simulink model "CS_SKILL_5_TDM"  (R2024a)
settings: Solver=VariableStepAuto  StartTime=0.0  StopTime=10.0  RelTol=1e-3
model workspace (MAT data in the model file):
  pi = 2
libraries: dspfdesign x3
settings Model: Creator=dev22  LastModifiedBy=dev22
settings RTWCC: GPUComputeCapability=3.5

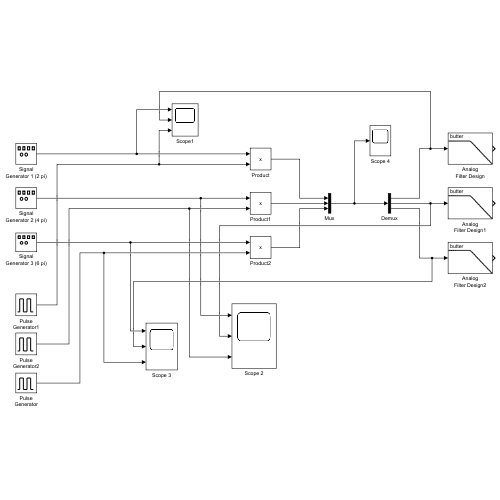
[thumbnail: Simulink's stored preview of the top-level diagram]
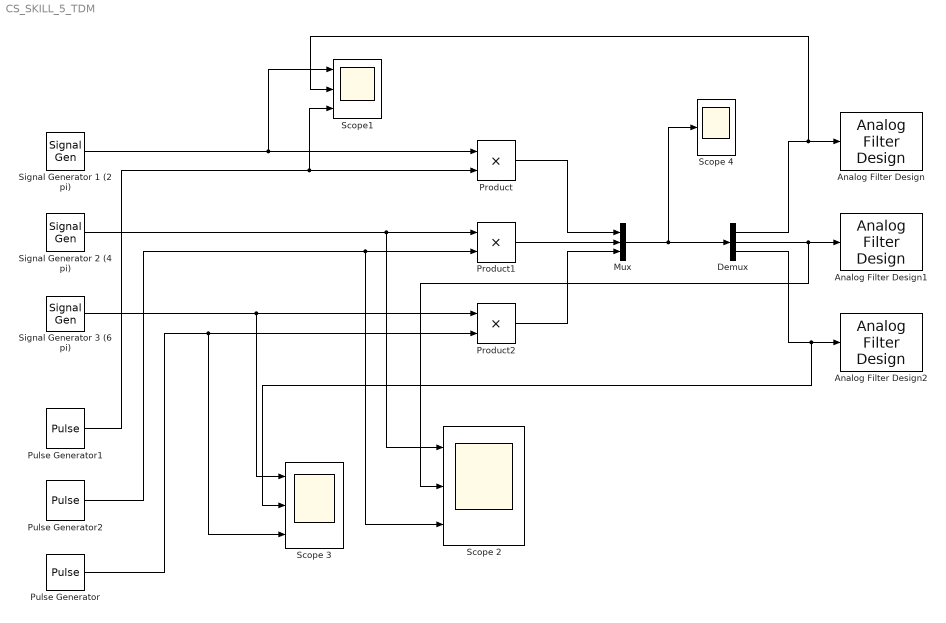
== system CS_SKILL_5_TDM ==
  Analog Filter Design : dspfdesign/Analog Filter Design  method=Butterworth  filttype=Lowpass  N=8  Wlo=2  Whi=80  Rp=2  Rs=40
  Analog Filter Design1 : dspfdesign/Analog Filter Design  method=Butterworth  filttype=Lowpass  N=8  Wlo=4  Whi=80  Rp=2  Rs=40
  Analog Filter Design2 : dspfdesign/Analog Filter Design  method=Butterworth  filttype=Lowpass  N=8  Wlo=6  Whi=80  Rp=2  Rs=40
  Demux : Demux  Outputs=3
  Mux : Mux  Inputs=3
  Product : Product
  Product1 : Product
  Product2 : Product
  Pulse Generator : DiscretePulseGenerator  PulseType=Time based  Period=0.1  PulseWidth=5  PhaseDelay=0.02
  Pulse Generator1 : DiscretePulseGenerator  PulseType=Time based  Period=0.1  PulseWidth=5
  Pulse Generator2 : DiscretePulseGenerator  PulseType=Time based  Period=0.1  PulseWidth=5  PhaseDelay=0.01
  Scope 2 : Scope  NumInputPorts=3
  Scope 3 : Scope  NumInputPorts=3
  Scope 4 : Scope
  Scope1 : Scope  NumInputPorts=3
  Signal Generator 1 (2 pi) : SignalGenerator  Frequency=2  Units=rad/sec
  Signal Generator 2 (4 pi) : SignalGenerator  Frequency=4  Units=rad/sec
  Signal Generator 3 (6 pi) : SignalGenerator  Frequency=6  Units=rad/sec
  wires:
  Pulse Generator1/1 -> Scope1/3, Product/2
  Pulse Generator2/1 -> Scope 2/3, Product1/2
  Pulse Generator/1 -> Scope 3/3, Product2/2
  Signal Generator 1 (2 pi)/1 -> Scope1/1, Product/1
  Signal Generator 2 (4 pi)/1 -> Scope 2/1, Product1/1
  Signal Generator 3 (6 pi)/1 -> Scope 3/1, Product2/1
  Product/1 -> Mux/1
  Product1/1 -> Mux/2
  Product2/1 -> Mux/3
  Mux/1 -> Scope 4/1, Demux/1
  Demux/3 -> Scope 3/2, Analog Filter Design2/1
  Demux/2 -> Scope 2/2, Analog Filter Design1/1
  Demux/1 -> Scope1/2, Analog Filter Design/1
